simulink model "exp4_theta"  (R2024b)
settings: Solver=ode45  StartTime=0.0  StopTime=10  MaxStep=0.01  RelTol=1e-3
settings Model: Creator=1  LastModifiedBy=1

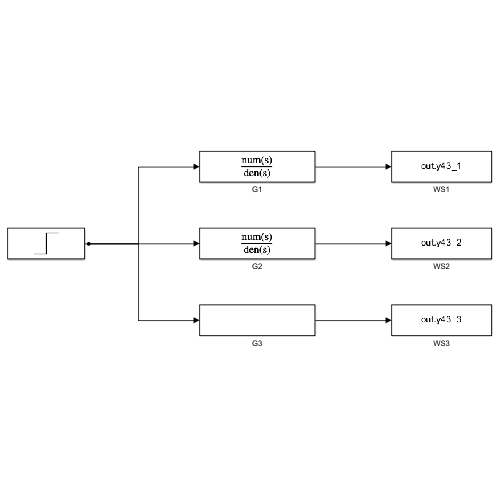
[thumbnail: Simulink's stored preview of the top-level diagram]
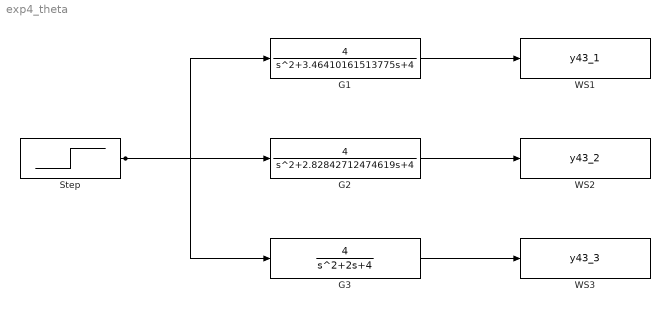
== system exp4_theta ==
  G1 : TransferFcn  Numerator=4  Denominator=[1 3.46410161513775 4]
  G2 : TransferFcn  Numerator=4  Denominator=[1 2.82842712474619 4]
  G3 : TransferFcn  Numerator=4  Denominator=[1 2 4]
  Step : Step  Time=0  After=2  SampleTime=0
  WS1 : ToWorkspace  VariableName=y43_1  SaveFormat=Timeseries  SampleTime=-1
  WS2 : ToWorkspace  VariableName=y43_2  SaveFormat=Timeseries  SampleTime=-1
  WS3 : ToWorkspace  VariableName=y43_3  SaveFormat=Timeseries  SampleTime=-1
  wires:
  Step/1 -> G1/1, G2/1, G3/1
  G1/1 -> WS1/1
  G2/1 -> WS2/1
  G3/1 -> WS3/1
